simulink model "designModel"  (R2021a)
settings: Solver=ode23  StartTime=0.0  StopTime=5  RelTol=1e-3  EnableMultiTasking=on
undefined symbols (not defined in the file or in its folder): Ion, Lithium
libraries: spsCurrentMeasurementLib x25, spsVoltageMeasurementLib x19, spsSeriesRLCBranchLib x11, spsGroundLib x6, powerlib_extras x4, dspsigops x3, spsPower3phInstantaneousLib x3, spsIGBTDiodeLib x2, spsUniversalBridgeLib x2, eeTotalHarmonicDistorsion x2, spsBatteryLib x1, spsParallelRLCBranchLib x1
(part 2 of 2)

== system designModel/Control Algorithm/Subsystem2/MSTF/Subsystem2/Subsystem ==
  a : Inport
  Constant : Constant  Value=314
  Gain : Gain  Gain=10
  Integrator : Integrator
  Integrator1 : Integrator
  Product : Product
  Product1 : Product
  Scope : Scope
  Sum : Sum  Inputs=-+
  Sum1 : Sum  Inputs=|+-
  a1 : Outport
  wires:
  Sum/1 -> Gain/1
  a/1 -> Sum/2
  Integrator/1 -> a1/1, Sum/1, Product/1
  Gain/1 -> Sum1/1
  Integrator1/1 -> Product1/1
  Sum1/1 -> Integrator/1
  Product/1 -> Integrator1/1
  Product1/1 -> Sum1/2
  Constant/1 -> Product1/2, Product/2, Scope/1

== system designModel/Control Algorithm/Subsystem2/MSTF/Subsystem2/Subsystem1 ==
  a : Inport
  Constant : Constant  Value=314
  Gain : Gain  Gain=10
  Integrator : Integrator
  Integrator1 : Integrator
  Product : Product
  Product1 : Product
  Scope : Scope
  Sum : Sum  Inputs=-+
  Sum1 : Sum  Inputs=|+-
  a1 : Outport
  wires:
  Sum/1 -> Gain/1
  a/1 -> Sum/2
  Integrator/1 -> a1/1, Sum/1, Product/1
  Gain/1 -> Sum1/1
  Integrator1/1 -> Product1/1
  Sum1/1 -> Integrator/1
  Product/1 -> Integrator1/1
  Product1/1 -> Sum1/2
  Constant/1 -> Product1/2, Product/2, Scope/1

== system designModel/Control Algorithm/Subsystem2/MSTF/Subsystem2/Subsystem2 ==
  a : Inport
  Constant : Constant  Value=314
  Gain : Gain  Gain=10
  Integrator : Integrator
  Integrator1 : Integrator
  Product : Product
  Product1 : Product
  Scope : Scope
  Sum : Sum  Inputs=-+
  Sum1 : Sum  Inputs=|+-
  a1 : Outport
  wires:
  Sum/1 -> Gain/1
  a/1 -> Sum/2
  Integrator/1 -> a1/1, Sum/1, Product/1
  Gain/1 -> Sum1/1
  Integrator1/1 -> Product1/1
  Sum1/1 -> Integrator/1
  Product/1 -> Integrator1/1
  Product1/1 -> Sum1/2
  Constant/1 -> Product1/2, Product/2, Scope/1

== matlab function designModel/MPPT ==
  settings: updateMethod=DISCRETE  sampleTime=1e-4
  data: tv input; Ipvin input; Vpvin input; Ipvin1 input; Vpvin1 input; Vdcref output; Vdcrefold input
function Vdcref = fcn(tv,Ipvin,Vpvin,Ipvin1,Vpvin1,Vdcrefold)
%#codegen
delVdc=0.2;
a=10;
delVpv=Vpvin-Vpvin1;
delIpv=Ipvin-Ipvin1;
if(tv>=0.6)
if(delVpv==0)
    if(delIpv==0)
        Vdcrefnew=Vdcrefold;
    else
        if(delIpv>0)
            Vdcrefnew=Vdcrefold-(delIpv/delVpv)*a;
    else
        Vdcrefnew=Vdcrefold+(delIpv/delVpv)*a;
        end
    end
    else
        if(delIpv/delVpv==-Ipvin/Vpvin)
            Vdcrefnew=Vdcrefold;
        else
            if(delIpv/delVpv>-Ipvin/Vpvin)
                Vdcrefnew=Vdcrefold-(delIpv/delVpv)*a;
            else
                Vdcrefnew=Vdcrefold+(delIpv/delVpv)*a;
            end
        end
end
Vdcref=Vdcrefnew;
else
Vdcref=810;
end


%Vdcref=658;
